simulink model "LH2_prop_valve_tuner"  (R2024b)
settings: Solver=ode15s  StartTime=0.0  StopTime=200  RelTol=1e-3
settings Model: Creator=MW  LastModifiedBy=MW

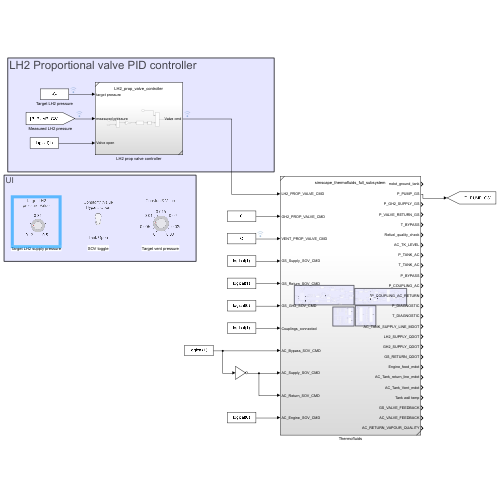
[thumbnail: Simulink's stored preview of the top-level diagram]
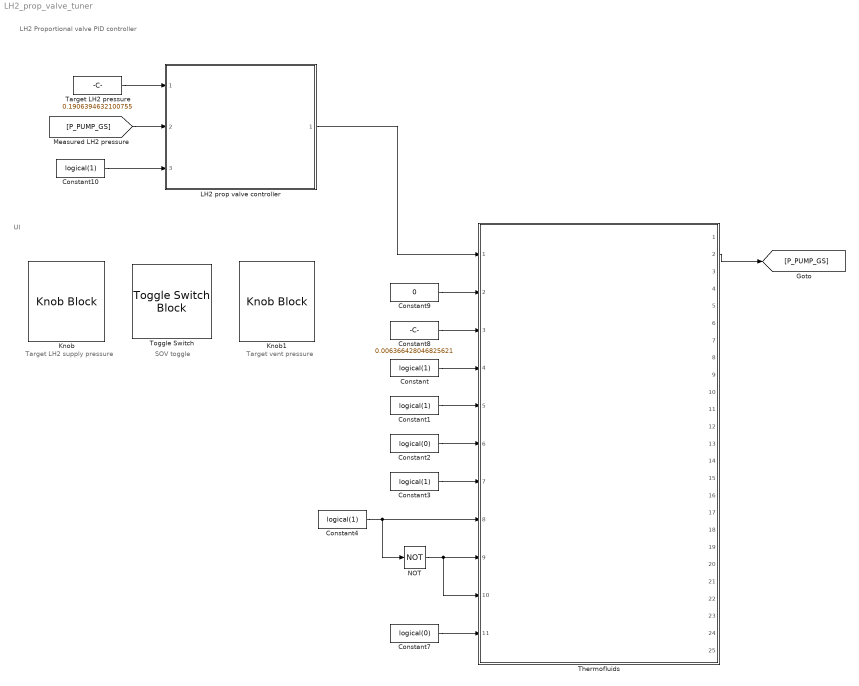
== system LH2_prop_valve_tuner ==
  note: Target LH2 supply pressure
  note: UI
  note: LH2 Proportional valve PID controller
  note: Target vent pressure
  note: SOV toggle
  Constant{,1,3..4,10} (5 alike) : Constant  Value=logical(1)
  Constant2 : Constant  Value=logical(0)
  Constant7 : Constant  Value=logical(0)
  Constant8 : Constant  Value=0.006366428046825621
  Constant9 : Constant  Value=0
  Knob : KnobBlock  ScaleMin=0.12  ScaleMax=0.5
  Knob1 : KnobBlock  ScaleMax=0.03
  LH2 prop valve controller : Subsystem  ReferencedSubsystem=LH2_prop_valve_controller
  NOT : Logic  Operator=NOT  IconShape=distinctive  AllPortsSameDT=off  OutDataTypeStr=boolean
  Target LH2 pressure : Constant  Value=0.1906394632100755
  Thermofluids : Subsystem  ReferencedSubsystem=simscape_thermofluids_full_subsystem
  Toggle Switch : ToggleSwitchBlock
      settings: Values={{'Tank Open', 'Bypass Open'}, [0 1]}
  wires:
  Constant/1 -> Thermofluids/4
  Constant1/1 -> Thermofluids/5
  Constant2/1 -> Thermofluids/6
  Constant3/1 -> Thermofluids/7
  Constant4/1 -> NOT/1, Thermofluids/8
  NOT/1 -> Thermofluids/9, Thermofluids/10
  Constant7/1 -> Thermofluids/11
  Constant8/1 -> Thermofluids/3
  Constant9/1 -> Thermofluids/2
  Target LH2 pressure/1 -> LH2 prop valve controller/1
  LH2 prop valve controller/1 -> Thermofluids/1
  Constant10/1 -> LH2 prop valve controller/3
  [P_PUMP_GS] -> LH2 prop valve controller/2
  Thermofluids/2 -> [P_PUMP_GS]
